simulink model "Quadcopter_Orientation_Altitude_Final_KCC_2023a"  (R2023a)
settings: Solver=ode5  StartTime=0.0  StopTime=6  FixedStep=0.0001  RelTol=1e-3  EnableMultiTasking=on
settings Model: Creator=craigk  LastModifiedBy=Admin
settings SolverCC: AlgebraicLoopSolver=TrustRegion
settings DataIOCC: SaveFormat=Array  ReturnWorkspaceOutputs=off
settings OptimizationCC: LifeSpan=inf
settings DebuggingCC: SolverPrmCheckMsg=warning  UnconnectedInputMsg=warning  UnconnectedOutputMsg=warning  UnconnectedLineMsg=warning  SFUnexpectedBacktrackingDiag=warning  SFNoUnconditionalDefaultTransitionDiag=warning  SFExecutionAtInitializationDiag=none  ArithmeticOperatorsInVariantConditions=warning
settings HardwareCC: ProdBitPerPointer=32  ProdBitPerSizeT=32  ProdBitPerPtrDiffT=32  ProdLargestAtomicFloat=None  ProdIntDivRoundTo=Undefined  ProdEndianess=Unspecified  ProdWordSize=32  ProdHWDeviceType=32-bit Generic
settings ModelReferenceCC: EnableRefExpFcnMdlSchedulingChecks=on  PropagateSignalLabelsOutOfModel=off
settings SFSimCC: SimUseLocalCustomCode=off  CustomCodeUndefinedFunction=UseInterfaceOnly
settings RTWCC: RTWUseLocalCustomCode=off  DLArmComputeVersion=19.05
settings CodeAppCC: StateflowObjectComments=on
settings GRTTargetCC: TargetLangStandard=C89/C90 (ANSI)
settings ConfigComp: CovMetricSettings=dw  CovSaveCumulativeToWorkspaceVar=on  CovSaveSingleToWorkspaceVar=on  CovExternalEMLEnable=off  CovSFcnEnable=off

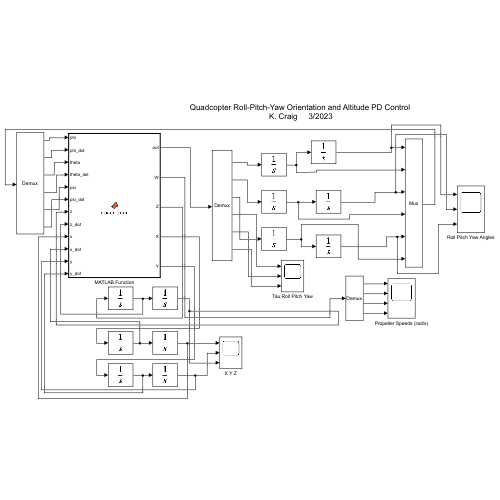
[thumbnail: Simulink's stored preview of the top-level diagram]
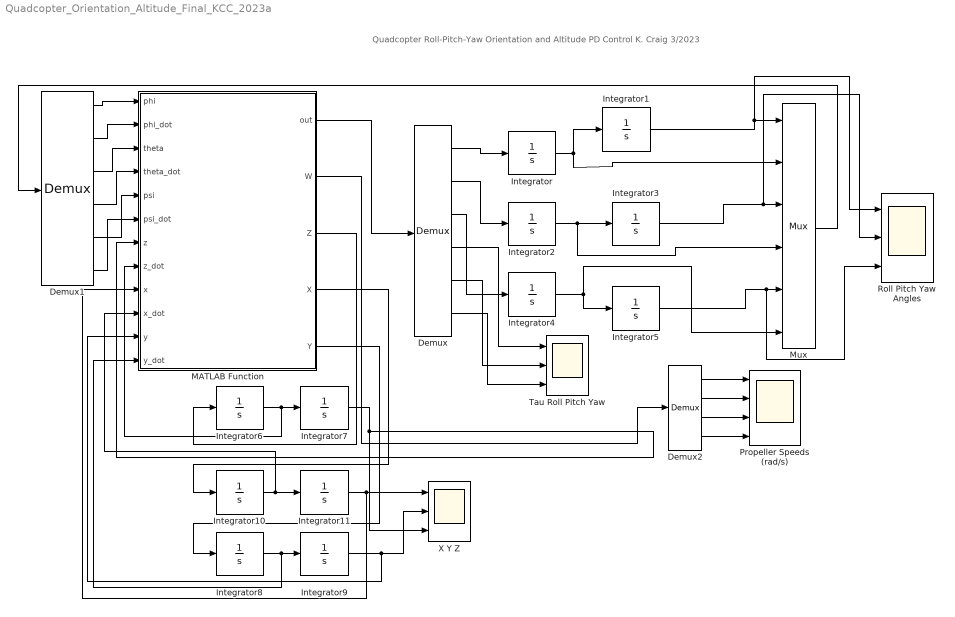
== system Quadcopter_Orientation_Altitude_Final_KCC_2023a ==
  note: Quadcopter Roll-Pitch-Yaw Orientation and Altitude PD Control
      | K. Craig 3/2023
  Demux : Demux  Outputs=6
      settings: DisplayOption=none
  Demux1 : Demux  Outputs=6
      settings: DisplayOption=none
  Demux2 : Demux
      settings: DisplayOption=none
  Integrator{,2,4,6,8..11} (8 alike) : Integrator
  Integrator1 : Integrator  InitialCondition=0.1745
  Integrator3 : Integrator  InitialCondition=0.1745
  Integrator5 : Integrator  InitialCondition=0.1745
  Integrator7 : Integrator  InitialCondition=1
  MATLAB Function : MATLAB Function  TreatAsAtomicUnit=on
  Mux : Mux  Inputs=6
  Propeller Speeds (rad/s) : Scope  NumInputPorts=4
  Roll Pitch Yaw Angles : Scope  NumInputPorts=3
  Tau Roll Pitch Yaw : Scope  NumInputPorts=3
  X Y Z : Scope  NumInputPorts=3
  wires:
  Integrator/1 -> Mux/2, Integrator1/1
  Integrator1/1 -> Roll Pitch Yaw Angles/1, Mux/1
  Integrator2/1 -> Mux/4, Integrator3/1
  Integrator3/1 -> Roll Pitch Yaw Angles/2, Mux/3
  Demux/1 -> Integrator/1
  MATLAB Function/1(out) -> Demux/1
  Demux/2 -> Integrator2/1
  Integrator5/1 -> Roll Pitch Yaw Angles/3, Mux/5
  Integrator4/1 -> Integrator5/1, Mux/6
  Demux/3 -> Integrator4/1
  Demux1/1 -> MATLAB Function/1(phi)
  Demux1/2 -> MATLAB Function/2(phi_dot)
  Demux1/3 -> MATLAB Function/3(theta)
  Demux1/4 -> MATLAB Function/4(theta_dot)
  Demux1/5 -> MATLAB Function/5(psi)
  Demux1/6 -> MATLAB Function/6(psi_dot)
  Mux/1 -> Demux1/1
  Demux/4 -> Tau Roll Pitch Yaw/1
  Demux/5 -> Tau Roll Pitch Yaw/2
  Demux/6 -> Tau Roll Pitch Yaw/3
  MATLAB Function/2(W) -> Demux2/1
  Demux2/1 -> Propeller Speeds (rad/s)/1
  Demux2/2 -> Propeller Speeds (rad/s)/2
  Demux2/3 -> Propeller Speeds (rad/s)/3
  Demux2/4 -> Propeller Speeds (rad/s)/4
  Integrator6/1 -> MATLAB Function/8(z_dot), Integrator7/1
  Integrator7/1 -> X Y Z/3, MATLAB Function/7(z)
  MATLAB Function/3(Z) -> Integrator6/1
  Integrator8/1 -> MATLAB Function/12(y_dot), Integrator9/1
  Integrator10/1 -> MATLAB Function/10(x_dot), Integrator11/1
  Integrator11/1 -> MATLAB Function/9(x), X Y Z/1
  Integrator9/1 -> X Y Z/2, MATLAB Function/11(y)
  MATLAB Function/4(X) -> Integrator10/1
  MATLAB Function/5(Y) -> Integrator8/1

== matlab function Quadcopter_Orientation_Altitude_Final_KCC_2023a/MATLAB Function ==
  data: phi input; out output; phi_dot input; theta input; theta_dot input; psi input; psi_dot input; W output; z input; z_dot input; Z output; x input; x_dot input; y input; y_dot input; X output; Y output
function [out,W,Z,X,Y] = quadcopter(phi, phi_dot, theta,...
    theta_dot, psi, psi_dot, z, z_dot, x, x_dot, y, y_dot )

% Quadcopter Parameters (SI Units)
Ix = 4.856E-3;
Iy = 4.856E-3;
Iz = 8.801E-3;
m = 0.468;
l = 0.225;
g = 9.81;
k = 2.980E-6;
b = 1.140E-7;
Ax = 0.25;
Ay = 0.25;
Az = 0.25;

% PD Control Gains
K_z_d = 2.5;
K_z_p = 1.5;
K_phi_d = 1.75;
K_theta_d = 1.75;
K_psi_d = 1.75;
K_phi_p = 6;
K_theta_p = 6;
K_psi_p = 6;

% Roll, Pitch and Yaw Position and Rate Commands
phi_dot_com = 0;
theta_dot_com = 0;
psi_dot_com = 0;
z_dot_com = 0;
phi_com = 0;
theta_com = 0;
psi_com = 0;
z_com = 0;

% Roll, Pitch, and Yaw Torques
tau_phi = Ix*(K_phi_d*(phi_dot_com - phi_dot) + K_phi_p*(phi_com - phi));
tau_theta = Iy*(K_theta_d*(theta_dot_com - theta_dot) + K_theta_p*(theta_com - theta));
tau_psi = Iz*(K_psi_d*(psi_dot_com - psi_dot) + K_psi_p*(psi_com - psi));

T = (g + K_z_d*(z_dot_com - z_dot) + K_z_p*(z_com -  z))*(m/(cos(phi)*cos(theta)));
w1 = (T/(4*k) - tau_theta/(2*k*l) - tau_psi/(4*b))^0.5;
w2 = (T/(4*k) - tau_phi/(2*k*l) + tau_psi/(4*b))^0.5;
w3 = (T/(4*k) + tau_theta/(2*k*l) - tau_psi/(4*b))^0.5;
w4 = (T/(4*k) + tau_phi/(2*k*l) + tau_psi/(4*b))^0.5;

% eta =[phi theta psi]'
% J*eta_ddot + C*eta_dot = [tau_phi tau_theta tau_psi]'

J = zeros(3,3);
C = zeros(3,3);

J(1,1) = Ix;
J(1,2) = 0;
J(1,3) = -Ix*sin(theta);
J(2,1) = 0;
J(2,2) = Iy*(cos(phi))^2 + Iz*(sin(phi))^2;
J(2,3) = (Iy-Iz)*cos(phi)*sin(phi)*cos(theta);
J(3,1) = -Ix*sin(theta);
J(3,2) = (Iy-Iz)*cos(phi)*sin(phi)*cos(theta);
J(3,3) = Ix*(sin(theta))^2 + Iy*(sin(phi))^2*(cos(theta))^2 + Iz*(cos(phi))^2*(cos(theta))^2;

C(1,1) = 0;
C(1,2) = (Iy-Iz)*(theta_dot*cos(phi)*sin(phi)+psi_dot*(sin(phi))^2*cos(theta))+...
    (Iz-Iy)*psi_dot*(cos(phi))^2*cos(theta)-Ix*psi_dot*cos(theta);
C(1,3) = (Iz-Iy)*psi_dot*cos(phi)*sin(phi)*(cos(theta))^2;
C(2,1) =  (Iz-Iy)*(theta_dot*cos(phi)*sin(phi)+psi_dot*sin(phi)*cos(theta))+...
    (Iy-Iz)*psi_dot*(cos(phi))^2*cos(theta)+Ix*psi_dot*cos(theta);
C(2,2) = (Iz-Iy)*phi_dot*cos(phi)*sin(phi);
C(2,3) = -Ix*psi_dot*sin(theta)*cos(theta)+Iy*psi_dot*(sin(phi))^2*sin(theta)*cos(theta)+...
    Iz*psi_dot*(cos(phi))^2*sin(theta)*cos(theta);
C(3,1) = (Iy-Iz)*psi_dot*(cos(theta))^2*sin(phi)*cos(phi)-Ix*theta_dot*cos(theta);
C(3,2) = (Iz-Iy)*(theta_dot*cos(phi)*sin(phi)*sin(theta)+phi_dot*(sin(phi))^2*cos(theta))+...
    (Iy-Iz)*phi_dot*(cos(phi))^2*cos(theta)+Ix*psi_dot*sin(theta)*cos(theta)-...
    Iy*psi_dot*(sin(phi))^2*sin(theta)*cos(theta)-Iz*psi_dot*(cos(phi))^2*sin(theta)*cos(theta);
C(3,3) = (Iy-Iz)*phi_dot*cos(phi)*sin(phi)*(cos(theta))^2-Iy*theta_dot*(sin(phi))^2*cos(theta)*sin(theta)-...
    Iz*theta_dot*(cos(phi))^2*cos(theta)*sin(theta)+Ix*theta_dot*cos(theta)*sin(theta);

B = [tau_phi tau_theta tau_psi]';

N = [phi_dot theta_dot psi_dot]';

W = [w1 w2 w3 w4];

z_ddot = (T/m)*(cos(phi)*cos(theta)) - g - (Az/m)*z_dot;
x_ddot = (T/m)*(sin(phi)*sin(psi)+cos(phi)*sin(theta)*cos(psi)) - (Ax/m)*x_dot;
y_ddot = (T/m)*(-sin(phi)*cos(psi)+cos(phi)*sin(theta)*sin(psi))- (Ay/m)*y_dot;

X = x_ddot;
Y = y_ddot;
Z = z_ddot;

out = [inv(J)*(B-C*N); B];
end
